simulink model "TFR_SchlittenPendel_test"  (R2020a)
settings: Solver=ode4  StartTime=0.0  StopTime=3.5  FixedStep=0.01  RelTol=1e-10
undefined symbols (not defined in the file or in its folder): simparams
libraries: dspfdesign x3
settings Model: Creator=Frederik  LastModifiedBy=Frederik

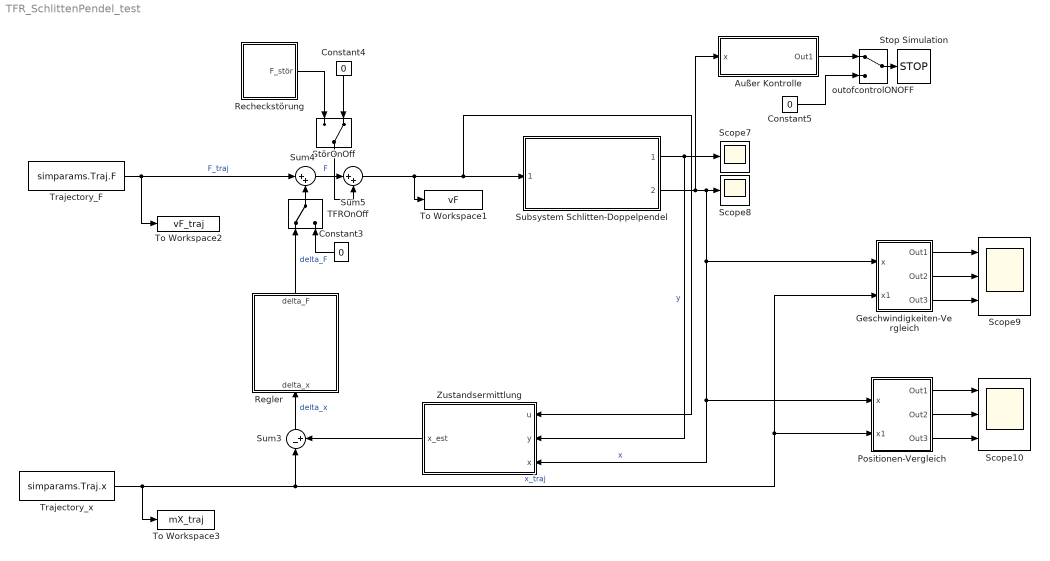
== system TFR_SchlittenPendel_test ==
  Außer Kontrolle : Subsystem
  Constant3 : Constant  Value=0
  Constant4 : Constant  Value=0
  Constant5 : Constant  Value=0
  Geschwindigkeiten-Vergleich : Subsystem
  Positionen-Vergleich : Subsystem
  Recheckstörung : Subsystem
  Regler : Subsystem  mask{RegData=simparams.TrajRegDataF}
      mask prompts: RegData "TrajRegDataF"
  Scope10 : Scope  NumInputPorts=3
  Scope7 : Scope
  Scope8 : Scope
  Scope9 : Scope  NumInputPorts=3
  Stop Simulation : Stop
  StörOnOff : ManualSwitch  CurrentSetting=0
  Subsystem Schlitten-Doppelpendel : Subsystem  ReferencedSubsystem=SchlittenPendel  params=simparams.gesamtmodell.schlittenpendel
  Sum3 : Sum  Inputs=|-+
  Sum4 : Sum  Inputs=|++
  Sum5 : Sum  Inputs=|++
  TFROnOff : ManualSwitch
  To Workspace1 : ToWorkspace  VariableName=vF  SaveFormat=Timeseries  SampleTime=-1
  To Workspace2 : ToWorkspace  VariableName=vF_traj  SaveFormat=Timeseries  SampleTime=-1
  To Workspace3 : ToWorkspace  VariableName=mX_traj  SaveFormat=Timeseries  SampleTime=-1
  Trajectory_F : FromWorkspace  VariableName=simparams.Traj.F  Interpolate=off  OutputAfterFinalValue=Setting to zero
  Trajectory_x : FromWorkspace  VariableName=simparams.Traj.x  Interpolate=off  OutputAfterFinalValue=Setting to zero
  Zustandsermittlung : Subsystem  Variant=on  VariantControl=Choice  PropagateVariantConditions=on  mask{BeoData=simparams.TrajRegDataF, xtype=Zustandsmessung}
      mask prompts: BeoData "Beobachter"; xtype "Zustandsermittlung"
      mask TypeOptions xtype: Zustandsmessung | Beobachter | Differenzieren
  outofcontrolONOFF : ManualSwitch
  wires:
  Außer Kontrolle/1(Out1) -> outofcontrolONOFF/1
  Positionen-Vergleich/2(Out2) -> Scope10/2
  Positionen-Vergleich/1(Out1) -> Scope10/1
  Regler/1(delta_F) -> TFROnOff/1  "delta_F"
  Geschwindigkeiten-Vergleich/3(Out3) -> Scope9/3
  StörOnOff/1 -> Sum5/2
  Subsystem Schlitten-Doppelpendel/2 -> Außer Kontrolle/1(x), Geschwindigkeiten-Vergleich/1(x), Zustandsermittlung/3(x), Positionen-Vergleich/1(x), Scope8/1  "x"
  Constant4/1 -> StörOnOff/2
  Geschwindigkeiten-Vergleich/2(Out2) -> Scope9/2
  Zustandsermittlung/1(x_est) -> Sum3/2
  Positionen-Vergleich/3(Out3) -> Scope10/3
  TFROnOff/1 -> Sum4/2
  Sum4/1 -> Sum5/1  "F"
  Trajectory_F/1 -> To Workspace2/1, Sum4/1  "F_traj"
  Recheckstörung/1(F_stör) -> StörOnOff/1
  Trajectory_x/1 -> Positionen-Vergleich/2(x1), Geschwindigkeiten-Vergleich/2(x1), Sum3/1, To Workspace3/1  "x_traj"
  Sum5/1 -> To Workspace1/1, Subsystem Schlitten-Doppelpendel/1, Zustandsermittlung/1(u)
  Subsystem Schlitten-Doppelpendel/1 -> Zustandsermittlung/2(y), Scope7/1  "y"
  Sum3/1 -> Regler/1(delta_x)  "delta_x"
  Constant3/1 -> TFROnOff/2
  Geschwindigkeiten-Vergleich/1(Out1) -> Scope9/1
  outofcontrolONOFF/1 -> Stop Simulation/1
  Constant5/1 -> outofcontrolONOFF/2

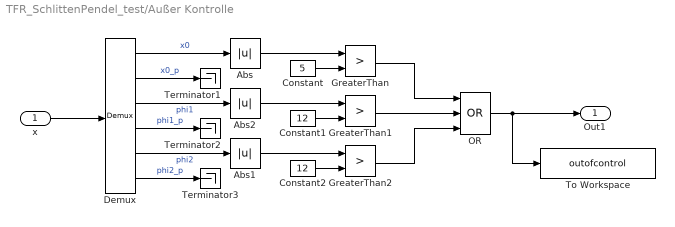
== system TFR_SchlittenPendel_test/Außer Kontrolle ==
  x : Inport
  Abs : Abs
  Abs1 : Abs
  Abs2 : Abs
  Constant : Constant  Value=5
  Constant1 : Constant  Value=12
  Constant2 : Constant  Value=12
  Demux : Demux  Outputs=6
  GreaterThan : RelationalOperator  Operator=>  OutDataTypeStr=boolean  RndMeth=Simplest
  GreaterThan1 : RelationalOperator  Operator=>  OutDataTypeStr=boolean  RndMeth=Simplest
  GreaterThan2 : RelationalOperator  Operator=>  OutDataTypeStr=boolean  RndMeth=Simplest
  OR : Logic  Operator=OR  Inputs=3  IconShape=distinctive  AllPortsSameDT=off  OutDataTypeStr=boolean
  Terminator1 : Terminator
  Terminator2 : Terminator
  Terminator3 : Terminator
  To Workspace : ToWorkspace  VariableName=outofcontrol  SaveFormat=Timeseries  SampleTime=-1
  Out1 : Outport
  wires:
  Constant/1 -> GreaterThan/2
  Demux/5 -> Abs1/1  "phi2"
  OR/1 -> To Workspace/1, Out1/1
  Demux/6 -> Terminator3/1  "phi2_p"
  Demux/4 -> Terminator2/1  "phi1_p"
  Abs2/1 -> GreaterThan1/1
  Abs/1 -> GreaterThan/1
  GreaterThan/1 -> OR/1
  GreaterThan1/1 -> OR/2
  Demux/2 -> Terminator1/1  "x0_p"
  Demux/3 -> Abs2/1  "phi1"
  Abs1/1 -> GreaterThan2/1
  Demux/1 -> Abs/1  "x0"
  GreaterThan2/1 -> OR/3
  Constant1/1 -> GreaterThan1/2
  Constant2/1 -> GreaterThan2/2
  x/1 -> Demux/1

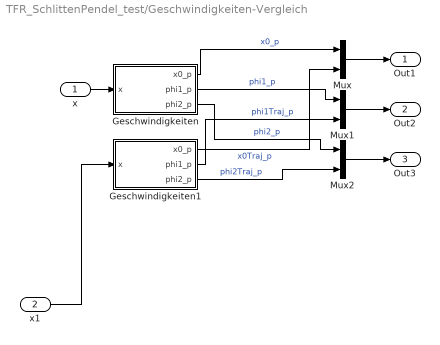
== system TFR_SchlittenPendel_test/Geschwindigkeiten-Vergleich ==
  x : Inport
  x1 : Inport  Port=2
  Geschwindigkeiten : Subsystem
  Geschwindigkeiten1 : Subsystem
  Mux : Mux  Inputs=2
  Mux1 : Mux  Inputs=2
  Mux2 : Mux  Inputs=2
  Out1 : Outport
  Out2 : Outport  Port=2
  Out3 : Outport  Port=3
  wires:
  Geschwindigkeiten/1(x0_p) -> Mux/1  "x0_p"
  x/1 -> Geschwindigkeiten/1(x)
  Mux1/1 -> Out2/1
  Geschwindigkeiten1/2(phi1_p) -> Mux1/2  "phi1Traj_p"
  Geschwindigkeiten/3(phi2_p) -> Mux2/1  "phi2_p"
  Geschwindigkeiten1/3(phi2_p) -> Mux2/2  "phi2Traj_p"
  x1/1 -> Geschwindigkeiten1/1(x)
  Mux2/1 -> Out3/1
  Geschwindigkeiten1/1(x0_p) -> Mux/2  "x0Traj_p"
  Geschwindigkeiten/2(phi1_p) -> Mux1/1  "phi1_p"
  Mux/1 -> Out1/1

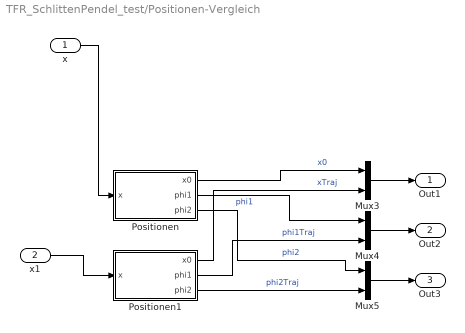
== system TFR_SchlittenPendel_test/Positionen-Vergleich ==
  x : Inport
  x1 : Inport  Port=2
  Mux3 : Mux  Inputs=2
  Mux4 : Mux  Inputs=2
  Mux5 : Mux  Inputs=2
  Positionen : Subsystem
  Positionen1 : Subsystem
  Out1 : Outport
  Out2 : Outport  Port=2
  Out3 : Outport  Port=3
  wires:
  Positionen/3(phi2) -> Mux5/1  "phi2"
  Mux3/1 -> Out1/1
  Positionen1/3(phi2) -> Mux5/2  "phi2Traj"
  x1/1 -> Positionen1/1(x)
  Mux5/1 -> Out3/1
  Mux4/1 -> Out2/1
  Positionen1/1(x0) -> Mux3/2  "xTraj"
  Positionen1/2(phi1) -> Mux4/2  "phi1Traj"
  Positionen/1(x0) -> Mux3/1  "x0"
  Positionen/2(phi1) -> Mux4/1  "phi1"
  x/1 -> Positionen/1(x)

== system TFR_SchlittenPendel_test/Recheckstörung ==
  Add : Sum  Inputs=+-
  Step : Step  Time=0.5  After=50  SampleTime=0
  Step2 : Step  After=50  SampleTime=0
  F_stör : Outport
  wires:
  Step/1 -> Add/1
  Step2/1 -> Add/2
  Add/1 -> F_stör/1

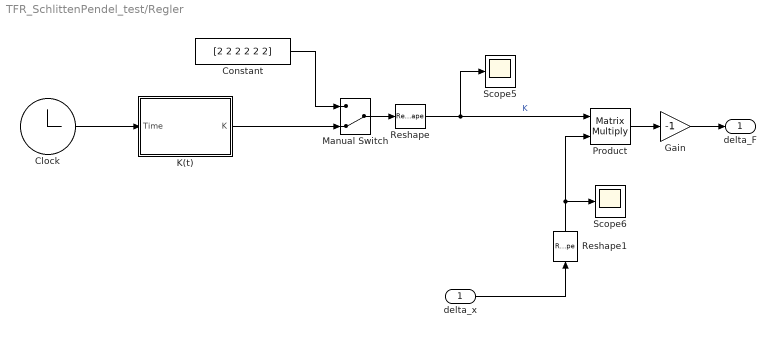
== system TFR_SchlittenPendel_test/Regler ==
  delta_x : Inport
  Clock : Clock
  Constant : Constant  Value=[2 2 2 2 2 2]
  Gain : Gain  Gain=-1
  K(t) : Subsystem
  Manual Switch : ManualSwitch  CurrentSetting=0
  Product : Product  Multiplication=Matrix(*)
  Reshape : Reshape  OutputDimensionality=Row vector (2-D)
  Reshape1 : Reshape  OutputDimensionality=Column vector (2-D)
  Scope5 : Scope
  Scope6 : Scope
  delta_F : Outport
  wires:
  Product/1 -> Gain/1
  Reshape1/1 -> Product/2, Scope6/1
  Reshape/1 -> Scope5/1, Product/1  "K"
  delta_x/1 -> Reshape1/1
  Constant/1 -> Manual Switch/1
  Gain/1 -> delta_F/1
  Manual Switch/1 -> Reshape/1
  Clock/1 -> K(t)/1(Time)
  K(t)/1(K) -> Manual Switch/2

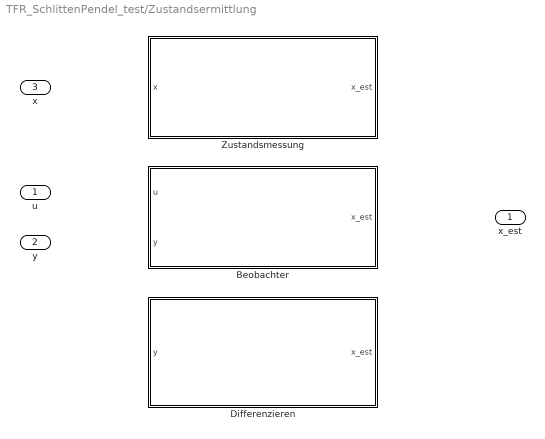
== system TFR_SchlittenPendel_test/Zustandsermittlung ==
  u : Inport
  y : Inport  Port=2
  x : Inport  Port=3
  Beobachter : Subsystem  VariantControl=simparams.Zustandsermittlung==2
  Differenzieren : Subsystem  VariantControl=simparams.Zustandsermittlung==3
  Zustandsmessung : Subsystem  VariantControl=simparams.Zustandsermittlung==1
  x_est : Outport

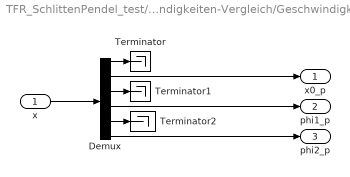
== system TFR_SchlittenPendel_test/Geschwindigkeiten-Vergleich/Geschwindigkeiten ==
  x : Inport
  Demux : Demux  Outputs=6
  Terminator : Terminator
  Terminator1 : Terminator
  Terminator2 : Terminator
  x0_p : Outport
  phi1_p : Outport  Port=2
  phi2_p : Outport  Port=3
  wires:
  Demux/4 -> phi1_p/1
  Demux/2 -> x0_p/1
  Demux/5 -> Terminator2/1
  x/1 -> Demux/1
  Demux/3 -> Terminator1/1
  Demux/1 -> Terminator/1
  Demux/6 -> phi2_p/1

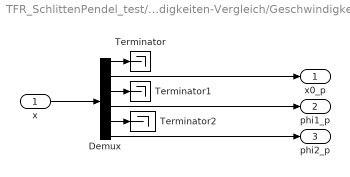
== system TFR_SchlittenPendel_test/Geschwindigkeiten-Vergleich/Geschwindigkeiten1 ==
  x : Inport
  Demux : Demux  Outputs=6
  Terminator : Terminator
  Terminator1 : Terminator
  Terminator2 : Terminator
  x0_p : Outport
  phi1_p : Outport  Port=2
  phi2_p : Outport  Port=3
  wires:
  Demux/4 -> phi1_p/1
  Demux/2 -> x0_p/1
  Demux/5 -> Terminator2/1
  x/1 -> Demux/1
  Demux/3 -> Terminator1/1
  Demux/1 -> Terminator/1
  Demux/6 -> phi2_p/1

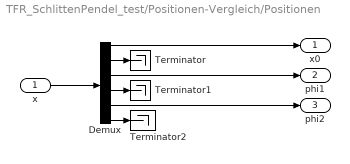
== system TFR_SchlittenPendel_test/Positionen-Vergleich/Positionen ==
  x : Inport
  Demux : Demux  Outputs=6
  Terminator : Terminator
  Terminator1 : Terminator
  Terminator2 : Terminator
  x0 : Outport
  phi1 : Outport  Port=2
  phi2 : Outport  Port=3
  wires:
  Demux/3 -> phi1/1
  Demux/1 -> x0/1
  x/1 -> Demux/1
  Demux/5 -> phi2/1
  Demux/2 -> Terminator/1
  Demux/4 -> Terminator1/1
  Demux/6 -> Terminator2/1

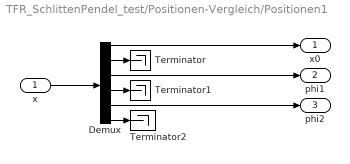
== system TFR_SchlittenPendel_test/Positionen-Vergleich/Positionen1 ==
  x : Inport
  Demux : Demux  Outputs=6
  Terminator : Terminator
  Terminator1 : Terminator
  Terminator2 : Terminator
  x0 : Outport
  phi1 : Outport  Port=2
  phi2 : Outport  Port=3
  wires:
  Demux/3 -> phi1/1
  Demux/1 -> x0/1
  x/1 -> Demux/1
  Demux/5 -> phi2/1
  Demux/2 -> Terminator/1
  Demux/4 -> Terminator1/1
  Demux/6 -> Terminator2/1

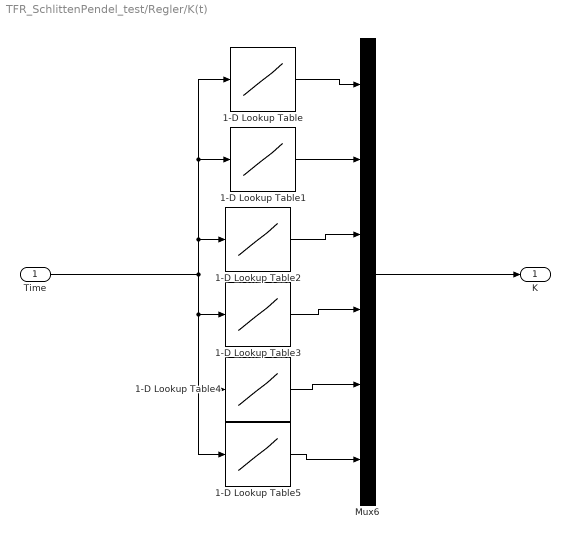
== system TFR_SchlittenPendel_test/Regler/K(t) ==
  Time : Inport
  1-D Lookup Table : Lookup_n-D  NumberOfTableDimensions=1  BreakpointsForDimension1=RegData.T.data  Table=RegData.K.data(:,1)  InternalRulePriority=Speed  RndMeth=Simplest  InputSameDT=on
  1-D Lookup Table1 : Lookup_n-D  NumberOfTableDimensions=1  BreakpointsForDimension1=RegData.T.data  Table=RegData.K.data(:,2)  InternalRulePriority=Speed  RndMeth=Simplest  InputSameDT=on
  1-D Lookup Table2 : Lookup_n-D  NumberOfTableDimensions=1  BreakpointsForDimension1=RegData.T.data  Table=RegData.K.data(:,3)  InternalRulePriority=Speed  RndMeth=Simplest  InputSameDT=on
  1-D Lookup Table3 : Lookup_n-D  NumberOfTableDimensions=1  BreakpointsForDimension1=RegData.T.data  Table=RegData.K.data(:,4)  InternalRulePriority=Speed  RndMeth=Simplest  InputSameDT=on
  1-D Lookup Table4 : Lookup_n-D  NumberOfTableDimensions=1  BreakpointsForDimension1=RegData.T.data  Table=RegData.K.data(:,5)  InternalRulePriority=Speed  RndMeth=Simplest  InputSameDT=on
  1-D Lookup Table5 : Lookup_n-D  NumberOfTableDimensions=1  BreakpointsForDimension1=RegData.T.data  Table=RegData.K.data(:,6)  InternalRulePriority=Speed  RndMeth=Simplest  InputSameDT=on
  Mux6 : Mux  Inputs=6
  K : Outport
  wires:
  1-D Lookup Table5/1 -> Mux6/6
  1-D Lookup Table2/1 -> Mux6/3
  1-D Lookup Table/1 -> Mux6/1
  Time/1 -> 1-D Lookup Table/1, 1-D Lookup Table1/1, 1-D Lookup Table2/1, 1-D Lookup Table5/1, 1-D Lookup Table4/1, 1-D Lookup Table3/1
  1-D Lookup Table4/1 -> Mux6/5
  1-D Lookup Table3/1 -> Mux6/4
  Mux6/1 -> K/1
  1-D Lookup Table1/1 -> Mux6/2

== system TFR_SchlittenPendel_test/Zustandsermittlung/Beobachter ==
  u : Inport
  y : Inport  Port=2
  Subsystem Reference : Subsystem  ReferencedSubsystem=Beobachter  A=BeoData.A.data  B=BeoData.B.data  C=BeoData.C.data  L=BeoData.L.data  xb0=BeoData.xb0
  x_est : Outport
  wires:
  Subsystem Reference/1 -> x_est/1
  y/1 -> Subsystem Reference/2
  u/1 -> Subsystem Reference/1

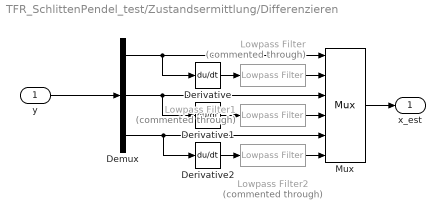
== system TFR_SchlittenPendel_test/Zustandsermittlung/Differenzieren ==
  y : Inport
  Demux : Demux  Outputs=3
  Derivative : Derivative  CoefficientInTFapproximation=1
  Derivative1 : Derivative  CoefficientInTFapproximation=1
  Derivative2 : Derivative  CoefficientInTFapproximation=1
  Lowpass Filter : dspfdesign/Lowpass Filter  Commented=through  FilterType=FIR  DesignForMinimumOrder=on  FilterOrder=50  PassbandFrequency=25  StopbandFrequency=100  PassbandRipple=0.1  StopbandAttenuation=80  InheritSampleRate=off  SampleRate=1000  SimulateUsing=Interpreted execution  roundingMode=Floor  coeffsDataTypeStr=fixdt(1,16)
  Lowpass Filter1 : dspfdesign/Lowpass Filter  Commented=through  FilterType=FIR  DesignForMinimumOrder=on  FilterOrder=50  PassbandFrequency=25  StopbandFrequency=100  PassbandRipple=0.1  StopbandAttenuation=80  InheritSampleRate=off  SampleRate=1000  SimulateUsing=Interpreted execution  roundingMode=Floor  coeffsDataTypeStr=fixdt(1,16)
  Lowpass Filter2 : dspfdesign/Lowpass Filter  Commented=through  FilterType=FIR  DesignForMinimumOrder=on  FilterOrder=50  PassbandFrequency=25  StopbandFrequency=100  PassbandRipple=0.1  StopbandAttenuation=80  InheritSampleRate=off  SampleRate=1000  SimulateUsing=Interpreted execution  roundingMode=Floor  coeffsDataTypeStr=fixdt(1,16)
  Mux : Mux  Inputs=6
  x_est : Outport
  wires:
  Mux/1 -> x_est/1
  y/1 -> Demux/1
  Demux/1 -> Derivative/1, Mux/1
  Demux/2 -> Derivative1/1, Mux/3
  Demux/3 -> Derivative2/1, Mux/5
  Derivative/1 -> Lowpass Filter/1
  Derivative1/1 -> Lowpass Filter1/1
  Derivative2/1 -> Lowpass Filter2/1
  Lowpass Filter/1 -> Mux/2
  Lowpass Filter1/1 -> Mux/4
  Lowpass Filter2/1 -> Mux/6

== system TFR_SchlittenPendel_test/Zustandsermittlung/Zustandsmessung ==
  x : Inport
  x_est : Outport
  wires:
  x/1 -> x_est/1
